simulink library "Wheels"  (R2015a)
settings: Solver=ode45  StartTime=0.0  StopTime=10.0  RelTol=1e-3
libraries: arduinodue_drivers x4, arduinolib x2
settings Model: Creator=tbaroche  LastModifiedBy=tbaroche

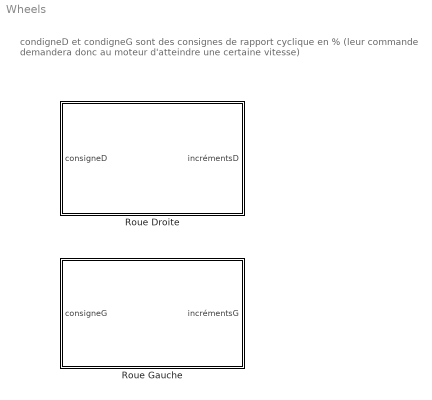
== system Wheels ==
  note: condigneD et condigneG sont des consignes de rapport cyclique en %
      | (leur commande demandera donc au moteur d'atteindre une certaine vitesse)
  Roue Droite : Subsystem
  Roue Gauche : Subsystem

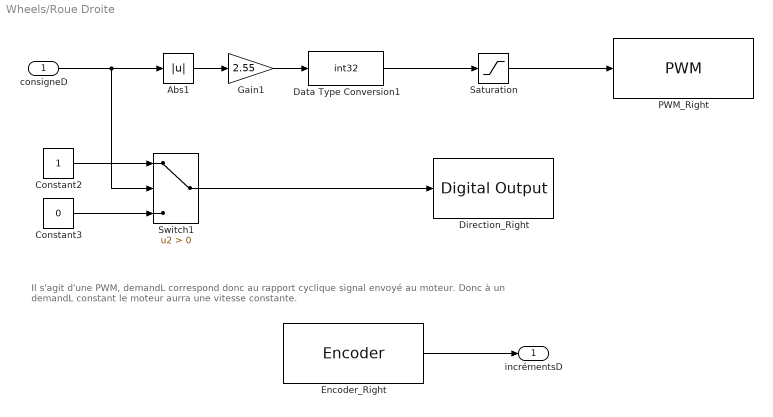
== system Wheels/Roue Droite ==
  note: Il s'agit d'une PWM, demandL correspond donc au rapport cyclique signal envoyé au moteur.
      | Donc à un demandL constant le moteur aurra une vitesse constante.
  consigneD : Inport  SampleTime=0
  Abs1 : Abs
  Constant2 : Constant  OutDataTypeStr=uint8
  Constant3 : Constant  Value=0  OutDataTypeStr=uint8
  Data Type Conversion1 : DataTypeConversion  OutDataTypeStr=int32  SaturateOnIntegerOverflow=on
  Direction_Right : arduinolib/Digital Output  pinNumber=4  blockPlatform=arduino
  Encoder_Right : arduinodue_drivers/Encoder  pinA=16  pinB=17
  Gain1 : Gain  Gain=2.55
  PWM_Right : arduinodue_drivers/PWM  pinNumber=5
  Saturation : Saturate  UpperLimit=255  LowerLimit=0
  Switch1 : Switch  Criteria=u2 > Threshold
  incrémentsD : Outport  OutDataTypeStr=int32
  wires:
  Data Type Conversion1/1 -> Saturation/1
  Gain1/1 -> Data Type Conversion1/1
  Abs1/1 -> Gain1/1
  Constant3/1 -> Switch1/3
  Saturation/1 -> PWM_Right/1
  Constant2/1 -> Switch1/1
  consigneD/1 -> Switch1/2, Abs1/1
  Encoder_Right/1 -> incrémentsD/1
  Switch1/1 -> Direction_Right/1

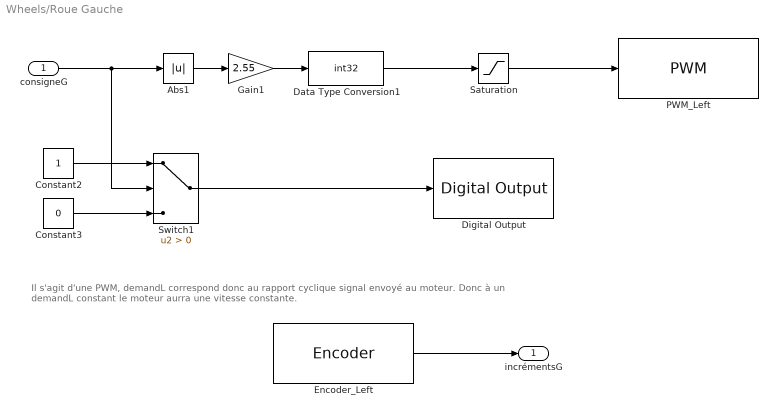
== system Wheels/Roue Gauche ==
  note: Il s'agit d'une PWM, demandL correspond donc au rapport cyclique signal envoyé au moteur.
      | Donc à un demandL constant le moteur aurra une vitesse constante.
  consigneG : Inport  SampleTime=0
  Abs1 : Abs
  Constant2 : Constant  OutDataTypeStr=uint8
  Constant3 : Constant  Value=0  OutDataTypeStr=uint8
  Data Type Conversion1 : DataTypeConversion  OutDataTypeStr=int32  SaturateOnIntegerOverflow=on
  Digital Output : arduinolib/Digital Output  pinNumber=7  blockPlatform=arduino
  Encoder_Left : arduinodue_drivers/Encoder  pinA=19  pinB=18
  Gain1 : Gain  Gain=2.55
  PWM_Left : arduinodue_drivers/PWM  pinNumber=6
  Saturation : Saturate  UpperLimit=255  LowerLimit=0
  Switch1 : Switch  Criteria=u2 > Threshold
  incrémentsG : Outport  OutDataTypeStr=int32
  wires:
  consigneG/1 -> Switch1/2, Abs1/1
  Switch1/1 -> Digital Output/1
  Constant3/1 -> Switch1/3
  Constant2/1 -> Switch1/1
  Saturation/1 -> PWM_Left/1
  Data Type Conversion1/1 -> Saturation/1
  Gain1/1 -> Data Type Conversion1/1
  Abs1/1 -> Gain1/1
  Encoder_Left/1 -> incrémentsG/1
